simulink model "3-phase transmission line simulink model"  (R2023b)
settings: Solver=VariableStepAuto  StartTime=0.0  StopTime=1  RelTol=1e-3
libraries: dspstat3 x4, spsPiSectionLineLib x3, spsThreePhaseVIMeasurementLib x2, spsThreePhaseSeriesRLCLoadLib x1, spsThreePhaseSourceLib x1, spspowerguiLib x1
settings Model: Creator=Rahul  LastModifiedBy=Rahul

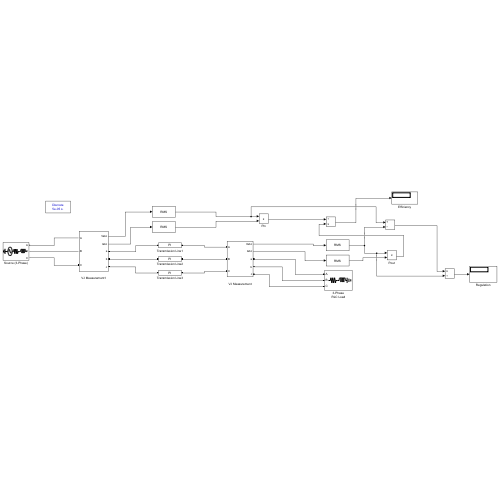
[thumbnail: Simulink's stored preview of the top-level diagram]
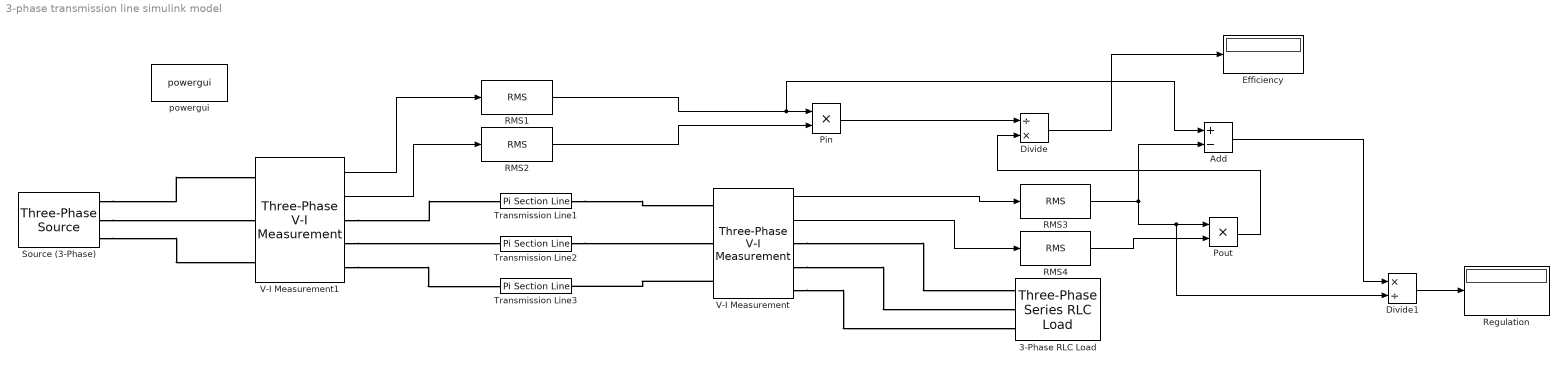
== system 3-phase transmission line simulink model ==
  " V-I Measurement" : spsThreePhaseVIMeasurementLib/Three-Phase V-I Measurement  VoltageMeasurement=phase-to-ground  SetLabelV=off  LabelV=Vabc  Vpu=off  VpuLL=off  CurrentMeasurement=yes  SetLabelI=off  LabelI=Iabc  Ipu=off  Pbase=100e6  Vbase=500e3  OutputType=Complex  PhasorSimulation=off  PSBequivalent=0
  " V-I Measurement1" : spsThreePhaseVIMeasurementLib/Three-Phase V-I Measurement  VoltageMeasurement=phase-to-ground  SetLabelV=off  LabelV=Vabc  Vpu=off  VpuLL=off  CurrentMeasurement=yes  SetLabelI=off  LabelI=Iabc  Ipu=off  Pbase=100e6  Vbase=500e3  OutputType=Complex  PhasorSimulation=off  PSBequivalent=0
  3-Phase RLC Load : spsThreePhaseSeriesRLCLoadLib/Three-Phase Series RLC Load  LConnTagsString=A|B|C  Configuration=Y (grounded)  NominalVoltage=400e3  Vabc=[1e3 1e3 1e3]  Vabcp=[1e3 1e3 1e3]  NominalFrequency=50  UnbalancedPower=off  ActivePower=495e6  InductivePower=857.36e6  CapacitivePower=0  Pabc=[10e3 9e3 11e3]  QLabc=[100 90 110]  QCabc=[100 90 110]  Pabcp=[10e3 9e3 11e3]  QLabcp=[100 90 110]  QCabcp=[100 90 110]  Measurements=None  LoadType=constant Z
  Add : Sum  Inputs=+-
  Divide : Product  Inputs=/*
  Divide1 : Product  Inputs=*/
  Efficiency : Display
  Pin : Product
  Pout : Product
  RMS{1..4} (4 alike) : dspstat3/RMS  run=off  directionMode=Each column  dimension=1  InputProcessing=Columns as channels (frame based)  reset_popup=None
  Regulation : Display
  Source (3-Phase) : spsThreePhaseSourceLib/Three-Phase Source  InternalConnection=Yg  VoltagePhases=off  Voltage=400e3  PhaseAngle=0  Voltage_phases=[25e3 25e3 25e3]/sqrt(3)  PhaseAngles_phases=[0 -120 +120]  Frequency=50  NonIdealSource=on  SpecifyImpedance=off  Resistance=0.8929  Inductance=16.58e-3  ShortCircuitLevel=100e6  BaseVoltage=25e3  XRratio=7  BusType=swing  Pref=10e3  Qref=0  Prefabc=[10e3, 10e3, 10e3]  Qrefabc=[0, 0, 0]  Qmin=-inf  Qmax=inf
  Transmission Line1 : spsPiSectionLineLib/Pi Section Line  LConnTagsString=1  RConnTagsString=1  Phases=1  PiSections=1  Length=160  Frequency=50  Resistance=0.642  Inductance=1.39e-3  Capacitance=1.296e-9  SpecifyConductance=off  Conductance=0  Measurements=None  Measurements2=None
      settings: LibrarySourceBlock=sps_lib/Power Grid Elements/Pi Section Line
  Transmission Line2 : spsPiSectionLineLib/Pi Section Line  LConnTagsString=1  RConnTagsString=1  Phases=1  PiSections=1  Length=160  Frequency=50  Resistance=0.642  Inductance=1.39e-3  Capacitance=1.296e-9  SpecifyConductance=off  Conductance=0  Measurements=None  Measurements2=None
      settings: LibrarySourceBlock=sps_lib/Power Grid Elements/Pi Section Line
  Transmission Line3 : spsPiSectionLineLib/Pi Section Line  LConnTagsString=1  RConnTagsString=1  Phases=1  PiSections=1  Length=160  Frequency=50  Resistance=0.642  Inductance=1.39e-3  Capacitance=1.296e-9  SpecifyConductance=off  Conductance=0  Measurements=None  Measurements2=None
      settings: LibrarySourceBlock=sps_lib/Power Grid Elements/Pi Section Line
  powergui : spspowerguiLib/powergui  Priority=1  SimulationMode=Discrete  SampleTime=50e-6  frequency=50  Iterations=50  frequencyindice=50  Pbase=100e6  ErrMax=1e-4  UnitsV=kV  UnitsW=MW  buscounter=0  FunctionMessages=off  echomessages=off  EnableUseOfTLC=off  CurrentSourceSwitches=off  DisableSnubberDevices=off  DisableRonSwitches=off  DisableVfSwitches=off  DisplayEquations=off  AutomaticDiscreteSolvers=off  SolverType=Tustin/Backward Euler (TBE)  Interpol=off  ExternalGateDelay=off  methode=off  Ts=100  x0status=blocks  SPID=on  SwTol=0  HookPort=off  NonlinearTolerance=1e-4  nMaxIteration=100  ContinueOnMaxIteration=off  RestoreLinks=warning  ResistiveCurrentMeasurement=off  Frange=[0:2:500]  Ylog=off  Xlog=on  ShowGrid=off  save=off  variable=ZData  structure=0  ZoomFFT=off  StartTime=0.0  cycles=1  DisplayStyle=1  fundamental=60  FreqAxis=off  MaxFrequency=1000  frequencyindicesteady=1  RmsSteady=1  display=off
  wires:
  " V-I Measurement1"/1 -> RMS1/1
  " V-I Measurement1"/2 -> RMS2/1
  Divide/1 -> Efficiency/1
  Add/1 -> Divide1/1
  Divide1/1 -> Regulation/1
  " V-I Measurement"/2 -> RMS4/1
  " V-I Measurement"/1 -> RMS3/1
  RMS1/1 -> Add/1, Pin/1
  RMS2/1 -> Pin/2
  RMS3/1 -> Divide1/2, Pout/1, Add/2
  RMS4/1 -> Pout/2
  Pin/1 -> Divide/1
  Pout/1 -> Divide/2
  connections:
  " V-I Measurement"/LConn3 -- Transmission Line3/RConn1
  Transmission Line2/RConn1 -- " V-I Measurement"/LConn2
  Transmission Line1/RConn1 -- " V-I Measurement"/LConn1
  " V-I Measurement"/RConn2 -- 3-Phase RLC Load/LConn2
  " V-I Measurement"/RConn3 -- 3-Phase RLC Load/LConn3
  " V-I Measurement1"/RConn2 -- Transmission Line2/LConn1
  " V-I Measurement1"/RConn1 -- Transmission Line1/LConn1
  " V-I Measurement1"/RConn3 -- Transmission Line3/LConn1
  Source (3-Phase)/RConn1 -- " V-I Measurement1"/LConn1
  Source (3-Phase)/RConn3 -- " V-I Measurement1"/LConn3
  Source (3-Phase)/RConn2 -- " V-I Measurement1"/LConn2
  " V-I Measurement"/RConn1 -- 3-Phase RLC Load/LConn1
